simulink model "PHIL_Experimentation"  (R2025a)
settings: Solver=FixedStepAuto  StartTime=0.0  StopTime=inf  FixedStep=0.0001  RelTol=1e-3
PostLoadFcn:
  | if any(exist('dsrtsu_mdlpostloadfcn', 'file') ~= 0), dsrtsu_mdlpostloadfcn('Execute', bdroot); end
InitFcn:
  | , if any(exist('rtifpga_mdlclblib', 'file') ~= 0), rtifpga_mdlclblib('Init', bdroot); end,
  | , if any(exist('dsmpb_private', 'file') ~= 0), dsmpb_private('dsmpb_mdlclblib', 'Init', bdroot); end,
undefined symbols (not defined in the file): G, GainI, GainVdc, OffsetI1, OffsetI2, OffsetVdc, T
libraries: dsmpblib x8
PreSaveFcn:
  | , if any(exist('dsmpb_private', 'file') ~= 0), dsmpb_private('dsmpb_mdlclblib', 'PreSave', bdroot); end,
CloseFcn:
  | , if any(exist('dsmpb_private', 'file') ~= 0), dsmpb_private('dsmpb_mdlclblib', 'Close', bdroot); end,
settings Model: DSMPB_ID_DATA={'132',struct('BlockId','c9eb2fc8-90ac-4e9b-9068-12357bfd6742','SignalIds',{{'6c23ef1c-e03d-4859-af71-2adc79b94187'}}),'23',struct('BlockId','3ebde5ff-2c0a-4178-a793-fcf709d724d1','SignalIds',{{'f27b2cf0-e2af-4dc6-9a19-a0c26cd001a4'}}),'42',struct('BlockId','49a58374-05d3-4ea8-acc0-1bfcf246a723','SignalIds',{{'0ef0f663-f70c-48c5-8b6b-4e283b0ccb28'}}),'63',struct('BlockId','915a77b0-0e55-4f3c-9cbf-97c5fe9b2d7e','SignalIds',{{'3b5ce7df-7de1-45ac-aabd-70b5ca045bb9','70a9fb95-1965-4781-aa79-78121be355a5','fa7b849d-74af-4bc8-b58a-104ff7ba60d7'}}),'72',struct('BlockId','d6c54500-ab9d-48f1-b1bd-f845a8eba63c','SignalIds',{{'c0b43ec9-4d08-4fbe-8262-9c39d2f7c85b'}}),'73',struct('BlockId','351f256b-03a9-411e-a474-5d404ada0f24','SignalIds',{{'81ce002f-1f4e-4239-af34-e879f97f29d3'}}),'74',struct('BlockId','7e575da0-a9dd-44f7-b1ee-b6a87fb307ba','SignalIds',{{'02e938a0-7677-4714-a2bf-9c904d011e37'}}),'85',struct('BlockId','3aa1295d-fd08-453a-93a8-5eb54c09410c','SignalIds',{{'e85d9f7b-b0f1-4e95-9ef4-54855227100f'}})}  DSRTSU_INTERNAL_RTIFPGA=220  DSRTSU_INTERNAL_RTISTBM_VER=25.1  Creator=e94179u  LastModifiedBy=e94179u
settings OptimizationCC: BlockReduction=off  ConditionallyExecuteInputs=off  OptimizeBlockIOStorage=off  BufferReuse=off
settings DebuggingCC: TasksWithSamePriorityMsg=none
settings HardwareCC: ProdBitPerLong=64.0  ProdLargestAtomicInteger=Integer  ProdWordSize=32.0  ProdLongLongMode=on  ProdHWDeviceType=Custom Processor->Custom
settings ModelReferenceCC: EnableParallelModelReferenceBuilds=on
settings RTWCC: SystemTargetFile=dsrt.tlc  GenCodeOnly=on  MakeCommand=make_dsrt  TemplateMakefile=dsrt_default_tmf  RTWVerbose=off  Description=dSPACE Target DSRT - Generates SIC files for import by ConfigurationDesk and VEOS. Provides code generation for Simulink models imported in ConfigurationDesk.
settings STFCustomTargetCC: SystemTargetFile=dsrt.tlc  TargetLangStandard=C99 (ISO)  MultiwordLength=2048.0  DynamicStringBufferSize=256.0  ParMdlRefBuildCompliant=on  GRTInterface=off  TRCGenerateDerivatives=off  TRCIsOmitVdOn=on  TRCGenerateStates=off  TRCOnlyGlobals=off  VDFType=TRC  TRCGenerateVirtualBlocks=off  TRCGenerateLabels=on  DSTargetArchitecture=Default  TRCGenerateParamValues=off
settings GRTTargetCC: CompOptLevelCompliant=off  ConcurrentExecutionCompliant=off  CombineOutputUpdateFcns=off  MatFileLogging=off  CPPClassGenCompliant=off  UseToolchainInfoCompliant=off

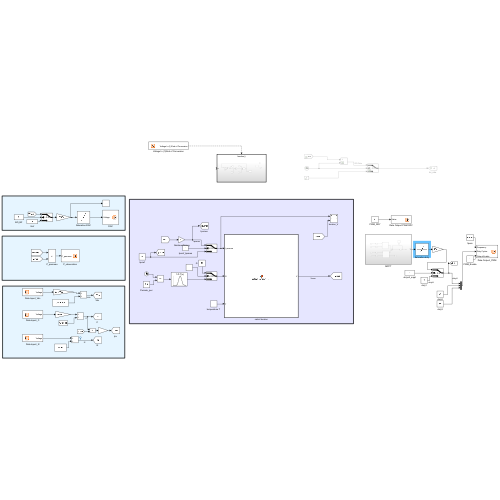
[thumbnail: Simulink's stored preview of the top-level diagram]
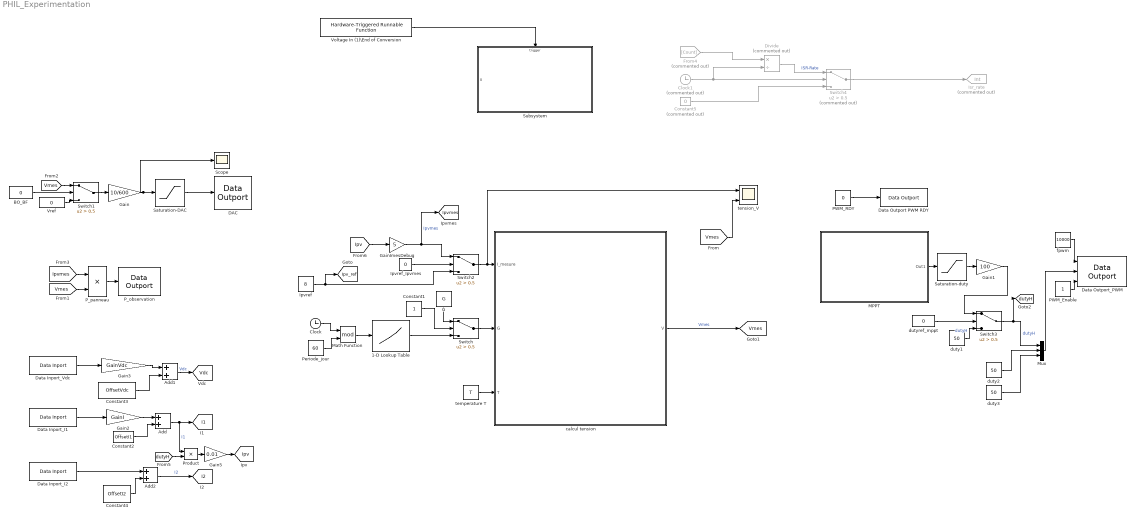
== system PHIL_Experimentation ==
  1-D Lookup Table : Lookup_n-D  NumberOfTableDimensions=1  BreakpointsForDimension1=[0 15 17.5 20 22.5 25 27.5 30 32.5 35 37.5 40 42.5 45 50 55 60]  Table=[0 0 50 150 350 600 850 1000 1100 1000 850 600 350 150 50 0 0]  ExtrapMethod=Clip  InternalRulePriority=Speed  RndMeth=Simplest
  Add : Sum
  Add1 : Sum
  Add2 : Sum
  BO_BF : Constant  Value=0
  Clock : Clock
  Clock1 : Clock  Commented=on
  Constant1 : Constant
  Constant2 : Constant  Value=OffsetI1
  Constant3 : Constant  Value=OffsetVdc
  Constant4 : Constant  Value=OffsetI2
  Constant5 : Constant  Commented=on  Value=0
  DAC : dsmpblib/Data Outport  Priority=-10000
      settings: SourceProductName=dSPACE Model Interface Package for Simulink (MIPS)
  Data Inport_I1 : dsmpblib/Data Inport  Priority=-10000
      settings: SourceProductName=dSPACE Model Interface Package for Simulink (MIPS)
  Data Inport_I2 : dsmpblib/Data Inport  Priority=-10000
      settings: SourceProductName=dSPACE Model Interface Package for Simulink (MIPS)
  Data Inport_Vdc : dsmpblib/Data Inport  Priority=10000
      settings: SourceProductName=dSPACE Model Interface Package for Simulink (MIPS)
  Data Outport PWM RDY : dsmpblib/Data Outport  Priority=-10000
      settings: SourceProductName=dSPACE Model Interface Package for Simulink (MIPS)
  Data Outport_PWM : dsmpblib/Data Outport  Priority=-10000
      settings: SourceProductName=dSPACE Model Interface Package for Simulink (MIPS)
  Divide : Product  Commented=on  Inputs=*/
  From4 : From  Commented=on  GotoTag=Count  TagVisibility=global
  G : Constant  Value=G
  Gain : Gain  Gain=10/600
  Gain1 : Gain  Gain=100
  Gain2 : Gain  Gain=GainI
  Gain3 : Gain  Gain=GainVdc
  Gain5 : Gain  Gain=0.01
  GainImesDebug : Gain  Gain=5
  Ipvref : Constant  Value=8
  Ipvref_Ipvmes : Constant  Value=0
  Isr_rate : Goto  Commented=on  GotoTag=Int  TagVisibility=global
  MPPT : Subsystem
  Math Function : Math  Operator=mod
  Mux : Mux  Inputs=3
  PWM_Enable : Constant
  PWM_RDY : Constant  Value=0
  P_observation : dsmpblib/Data Outport  Priority=-10000
      settings: SourceProductName=dSPACE Model Interface Package for Simulink (MIPS)
  P_panneau : Product
  Periode_jour : Constant  Value=60
  Product : Product
  Saturation-DAC : Saturate  UpperLimit=0.833  LowerLimit=0
  Saturation-duty : Saturate  UpperLimit=0.8  LowerLimit=0.2
  Scope : Scope
      settings: ActiveDisplayYMinimum=0.41621008700106643  ActiveDisplayYMaximum=0.620293115657243
  Subsystem : Subsystem
  Switch{,1..3} (4 alike) : Switch  Criteria=u2 > Threshold  Threshold=0.5  SaturateOnIntegerOverflow=off  InputSameDT=off
  Switch4 : Switch  Commented=on  Criteria=u2 > Threshold  Threshold=0.5  SaturateOnIntegerOverflow=off  InputSameDT=off
  Voltage In (1)\End of Conversion : dsmpblib/Hardware-Triggered Runnable Function
      settings: SourceProductName=dSPACE Model Interface Package for Simulink (MIPS)
  Vref : Constant  Value=0
  calcul tension : MATLAB Function  TreatAsAtomicUnit=on
  duty1 : Constant  Value=50
  duty2 : Constant  Value=50
  duty3 : Constant  Value=50
  dutyref_mppt : Constant  Value=0
  fpwm : Constant  Value=10000
  "temperature T " : Constant  Value=T
  "tension_V " : Scope  NumInputPorts=2
      settings: ActiveDisplayYMinimum=-18.219801940495174  ActiveDisplayYMaximum=42.151801144365422
  tag scope: I1=global, I2=global, Ipv=global, Ipv_ref=global, Ipvmes=global, Vdc=global, Vmes=global, dutyH=global
  wires:
  calcul tension/1(V) -> [Vmes]  "Vmes"
  P_panneau/1 -> P_observation/1
  [Ipvmes] -> P_panneau/1
  "temperature T "/1 -> calcul tension/3(T)
  [Vmes] -> P_panneau/2
  Switch/1 -> calcul tension/2(G)
  Gain/1 -> Saturation-DAC/1, Scope/1
  G/1 -> Switch/1
  1-D Lookup Table/1 -> Switch/3
  Constant1/1 -> Switch/2
  Periode_jour/1 -> Math Function/2
  Math Function/1 -> 1-D Lookup Table/1
  Clock/1 -> Math Function/1
  MPPT/1(Out1) -> Saturation-duty/1
  Constant2/1 -> Add/2
  Constant4/1 -> Add2/2
  Gain2/1 -> Add/1
  Data Inport_Vdc/1 -> Gain3/1
  Data Inport_I1/1 -> Gain2/1
  Gain3/1 -> Add1/1
  Constant3/1 -> Add1/2
  Add/1 -> Product/1, [I1]  "I1"
  Add1/1 -> [Vdc]  "Vdc"
  Add2/1 -> [I2]  "I2"
  Data Inport_I2/1 -> Add2/1
  Switch2/1 -> "tension_V "/1, calcul tension/1(I_mesure)
  PWM_RDY/1 -> Data Outport PWM RDY/1
  [Vmes] -> "tension_V "/2
  fpwm/1 -> Data Outport_PWM/1
  PWM_Enable/1 -> Data Outport_PWM/3
  Saturation-DAC/1 -> DAC/1
  Switch1/1 -> Gain/1
  Ipvref/1 -> [Ipv_ref], Switch2/3
  Switch3/1 -> [dutyH], Mux/1  "dutyH"
  Mux/1 -> Data Outport_PWM/2
  duty2/1 -> Mux/2
  duty3/1 -> Mux/3
  [Vmes] -> Switch1/1
  BO_BF/1 -> Switch1/2
  Vref/1 -> Switch1/3
  Ipvref_Ipvmes/1 -> Switch2/2
  GainImesDebug/1 -> [Ipvmes], Switch2/1  "Ipvmes"
  dutyref_mppt/1 -> Switch3/2
  duty1/1 -> Switch3/3  "dutyH"
  Gain1/1 -> Switch3/1
  [dutyH] -> Product/2
  Product/1 -> Gain5/1
  [Ipv] -> GainImesDebug/1
  Gain5/1 -> [Ipv]
  Voltage In (1)\End of Conversion/1 -> Subsystem/Trigger
  Clock1/1 -> Divide/2, Switch4/2
  Switch4/1 -> Isr_rate/1
  Constant5/1 -> Switch4/3
  Divide/1 -> Switch4/1  "ISR-Rate"
  From4/1 -> Divide/1
  Saturation-duty/1 -> Gain1/1

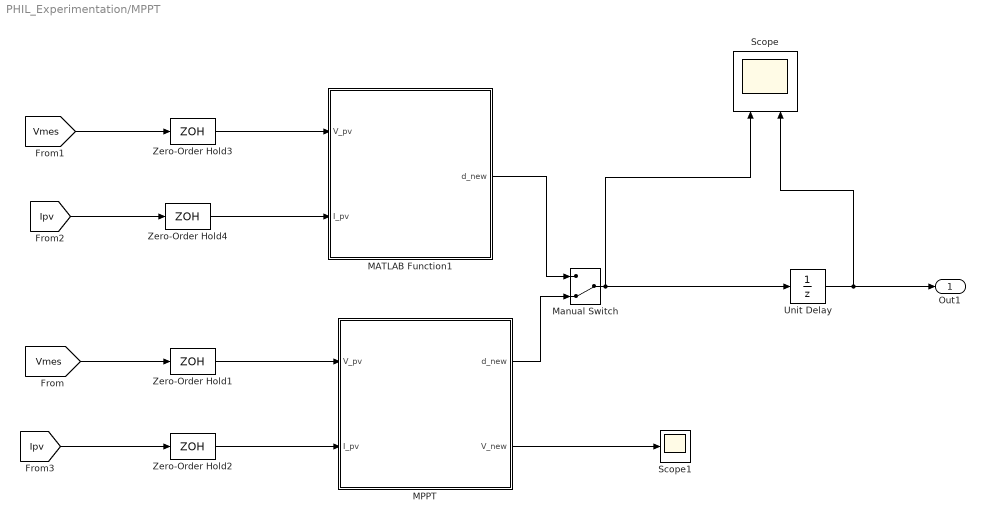
== system PHIL_Experimentation/MPPT ==
  MATLAB Function1 : MATLAB Function  TreatAsAtomicUnit=on
  MPPT : MATLAB Function  TreatAsAtomicUnit=on
  Manual Switch : ManualSwitch  CurrentSetting=0
  Scope : Scope  NumInputPorts=2
      settings: ActiveDisplayYMinimum=0.69625932381670541  ActiveDisplayYMaximum=0.84859620744849373  DataLoggingVariableName=ScopeData2
  Scope1 : Scope
      settings: DataLoggingVariableName=ScopeData3
  Unit Delay : UnitDelay  InitialCondition=0.4  SampleTime=-1  HasFrameUpgradeWarning=on
  Zero-Order Hold1 : ZeroOrderHold  SampleTime=0.1
  Zero-Order Hold2 : ZeroOrderHold  SampleTime=0.1
  Zero-Order Hold3 : ZeroOrderHold  SampleTime=0.001
  Zero-Order Hold4 : ZeroOrderHold  SampleTime=0.001
  Out1 : Outport
  wires:
  [Vmes] -> Zero-Order Hold1/1
  Unit Delay/1 -> Out1/1, Scope/2
  [Vmes] -> Zero-Order Hold3/1
  MPPT/1(d_new) -> Manual Switch/2
  MATLAB Function1/1(d_new) -> Manual Switch/1
  [Ipv] -> Zero-Order Hold2/1
  Manual Switch/1 -> Unit Delay/1, Scope/1
  [Ipv] -> Zero-Order Hold4/1
  MPPT/2(V_new) -> Scope1/1
  Zero-Order Hold1/1 -> MPPT/1(V_pv)
  Zero-Order Hold2/1 -> MPPT/2(I_pv)
  Zero-Order Hold3/1 -> MATLAB Function1/1(V_pv)
  Zero-Order Hold4/1 -> MATLAB Function1/2(I_pv)

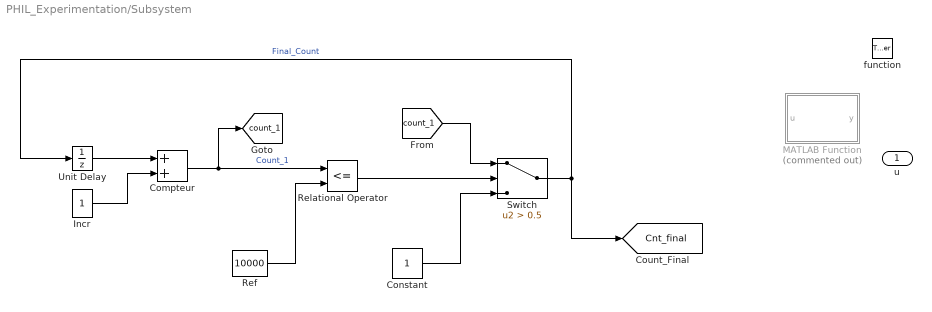
== system PHIL_Experimentation/Subsystem ==
  u : Inport
  function : TriggerPort  TriggerType=function-call  VariantControl=(inherit)
  Compteur : Sum
  Constant : Constant
  Incr : Constant
  MATLAB Function : MATLAB Function  Commented=on  TreatAsAtomicUnit=on
  Ref : Constant  Value=10000
  Relational Operator : RelationalOperator  Operator=<=  OutDataTypeStr=boolean  RndMeth=Simplest  InputSameDT=off
  Switch : Switch  Criteria=u2 > Threshold  Threshold=0.5  SaturateOnIntegerOverflow=off  InputSameDT=off
  Unit Delay : UnitDelay  SampleTime=-1  HasFrameUpgradeWarning=on
  tag scope: Cnt_final=global, count_1=global
  wires:
  Unit Delay/1 -> Compteur/1
  Incr/1 -> Compteur/2
  Ref/1 -> Relational Operator/2
  Compteur/1 -> Relational Operator/1, [count_1]  "Count_1"
  Relational Operator/1 -> Switch/2
  Constant/1 -> Switch/3
  [count_1] -> Switch/1
  Switch/1 -> Unit Delay/1, [Cnt_final]  "Final_Count"

== matlab function PHIL_Experimentation/MPPT/MPPT ==
  settings: updateMethod=DISCRETE  sampleTime=0.01
  data: V_pv input; I_pv input; d_new output; V_new output
function [d_new,V_new] = MPPT_intuitif(V_pv, I_pv)
    persistent V_old P_old
    
    if isempty(V_old)
        V_old = 20;     
        P_old = 0;
    end
    
    V_bus = 50;
    D = 0.0001;            
    
    % Puissance actuelle
    P_now = V_pv * I_pv;
    
    
    dP = P_now - P_old;
    dV = V_pv - V_old;
    
    
    if dP > 0
        if dV > 0
            V_new = V_pv + D;
        else
            V_new = V_pv - D;
        end
    else
        if dV < 0
            V_new = V_pv + D;
        else
            V_new = V_pv - D;
        end
    end
    
    % Sécurité sur V_new
    if V_new < 1
        V_new = 1;
    end
    if V_new > 36;
        V_new = 36;
    end
    
   
    d_new =  V_new/V_bus ;
    
    % Saturation duty
    if d_new < 0.1
        d_new = 0.1;
    end
    if d_new > 0.9
        d_new = 0.9;
    end
    
    % Mémorisation pour le prochain appel
    V_old = V_pv;
    P_old = P_now;
end

== matlab function PHIL_Experimentation/calcul tension ==
  data: I_mesure input; V output; G input; T input
function V = calcul_tension_NR(I_mesure, G, T)
   
    T = T + 273.15;
    
    Isc = 8.69;
    Voc = 0.61;       
    Ns = 60;
    k = 1.3806503e-23;
    q = 1.60217646e-19;
    a = 1.3;
    Rs = 0.04/60;
    Rp = 1271.1/60;
    Kv = -0.0038;
    Ki = 0.004;
    Gn = 1000;
    Tn = 298.15;
    
   
    dT = T - Tn;
    Vt = k*T/q;
    Io = (Isc + Ki*dT) / (exp(q*(Voc + Kv*dT)/(a*k*Tn)) - 1);
    Iph = (Isc + Ki*dT) * G/Gn;
    

    
    V = Voc; 
    for iter = 1:10  % 10 itérations 
        
        g = Iph - Io*(exp(q*(V + I_mesure*Rs)/(k*T*a)) - 1) ...
              - (V + I_mesure*Rs)/Rp - I_mesure;
        
        
        glin = -Io*(q/(k*T*a)) * exp(q*(V + I_mesure*Rs)/(k*T*a)) - 1/Rp;
        
       
        if abs(g) < 0.001
            break;
        end
        
      
        if glin ~= 0
            V = V - g/glin;
        else
            break;
        end
    end
    
    
    V = V * Ns;
    
   
    if V < 0
        V = 0;
    end
    if V > Voc * Ns
        V = Voc * Ns;
    end

    %if I_mesure > 8.5
        %I_mesure = 8.5;
    %end
end

== matlab function PHIL_Experimentation/MPPT/MATLAB Function1 ==
  settings: updateMethod=DISCRETE  sampleTime=0.01
  data: V_pv input; I_pv input; d_new output
function d_new = MPPT_Optimise(V_pv, I_pv)
    
    persistent V_ref V_old P_old
    
    if isempty(V_ref)
        V_ref = 20; 
        V_old = 20;     
        P_old = 0;
    end
    
    V_bus = 50;
    D = 0.1; 
    
    P_now = V_pv * I_pv;
    dP = P_now - P_old;
    dV = V_pv - V_old; 
    
    
    if dP > 0
        if dV > 0
            V_ref = V_ref + D;
        else
            V_ref = V_ref - D;
        end
    else
        if dV < 0
            V_ref = V_ref + D;
        else
            V_ref = V_ref - D;
        end
    end
    
    if V_ref < 10
        V_ref = 10;
    end
    if V_ref > 36
        V_ref = 36;
    end
    
    
    d_new =  V_ref/V_bus ;
    
    if d_new < 0.1
        d_new = 0.1;
    end
    if d_new > 0.9
        d_new = 0.9;
    end
    
    V_old = V_pv;
    P_old = P_now;
end

== matlab function PHIL_Experimentation/Subsystem/MATLAB Function ==
  data: u input; y output
function y = fcn(u)

y = u;
